simulink subsystem "Day3_Scenario_2"  (R2024a)
settings: Solver=VariableStepAuto  StartTime=0.0  StopTime=10.0  RelTol=1e-3
libraries: CarMaker4SL x8
settings Model: Creator=junhyung.cha  LastModifiedBy=User

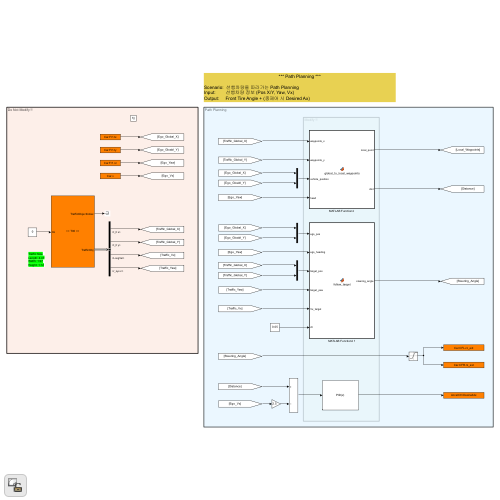
[thumbnail: Simulink's stored preview of the top-level diagram]
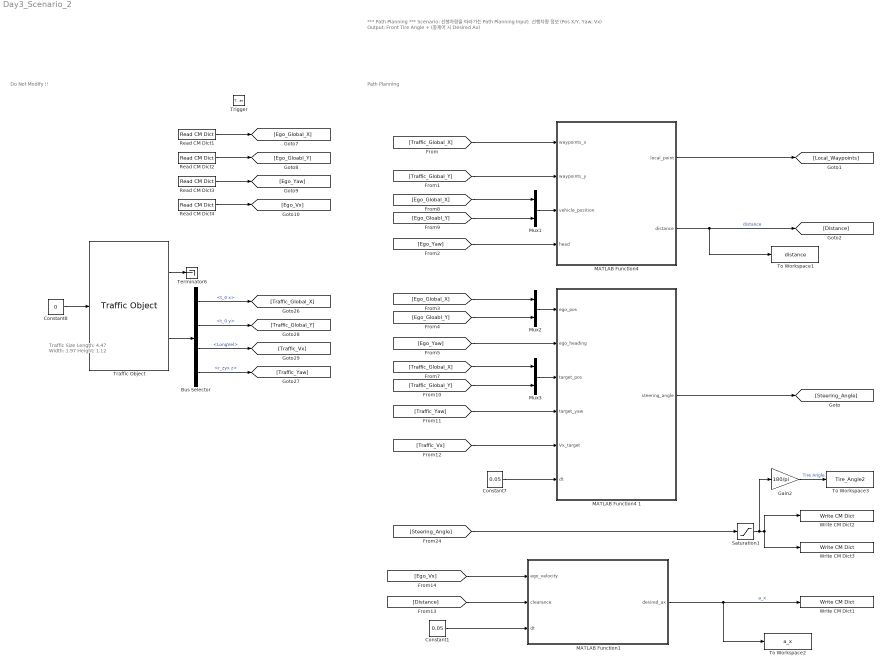
== system Day3_Scenario_2 ==
  note: Path Planning
  note: Do Not Modify !!
  note: *** Path Planning ***
      |
      | Scenario: 선행차량을 따라가는 Path Planning
      | Input: 선행차량 정보 (Pos X/Y, Yaw, Vx)
      | Output: Front Tire Angle + (종제어 시 Desired Ax)
  note: Traffic Size
      | Length: 4.47
      | Width: 1.97
      | Height: 1.12
  Trigger : TriggerPort  TriggerType=function-call  VariantControl=(inherit)
  Bus Selector : BusSelector  OutputSignals=t_0 x,t_0 y,LongVel,r_zyx z
  Constant1 : Constant  Value=0.05
  Constant7 : Constant  Value=0.05
  Constant8 : Constant  Value=0
  Gain2 : Gain  Gain=180/pi
  MATLAB Function1 : MATLAB Function  TreatAsAtomicUnit=on
  "MATLAB Function4 " : MATLAB Function  TreatAsAtomicUnit=on
  MATLAB Function4 1 : MATLAB Function  TreatAsAtomicUnit=on
  Mux1 : Mux  Inputs=2
  Mux2 : Mux  Inputs=2
  Mux3 : Mux  Inputs=2
  Read CM Dict1 : CarMaker4SL/Read CM Dict  xname=Car.Fr1.tx  xsync=off  xstime=Inherited
  Read CM Dict2 : CarMaker4SL/Read CM Dict  xname=Car.Fr1.ty  xsync=off  xstime=Inherited
  Read CM Dict3 : CarMaker4SL/Read CM Dict  xname=Car.Fr1.rz  xsync=off  xstime=Inherited
  Read CM Dict4 : CarMaker4SL/Read CM Dict  xname=Car.v  xsync=off  xstime=Inherited
  Saturation1 : Saturate  UpperLimit=pi/6  LowerLimit=-pi/6
  Terminator6 : Terminator
  To Workspace1 : ToWorkspace  VariableName=distance  SaveFormat=Timeseries  SampleTime=-1
  To Workspace2 : ToWorkspace  VariableName=a_x  SaveFormat=Timeseries  SampleTime=-1
  To Workspace3 : ToWorkspace  VariableName=Tire_Angle2  SaveFormat=Timeseries  SampleTime=-1
  Traffic Object : CarMaker4SL/Traffic Object  xname=T00  ximode=Traffic Id  xstime=Inherited
      settings: SourceProductName=CarMaker4SL
  Write CM Dict1 : CarMaker4SL/Write CM Dict  xname=AccelCtrl.DesiredAx  xsync=off
  Write CM Dict2 : CarMaker4SL/Write CM Dict  xname=Car.CFL.rz_ext  xsync=off
  Write CM Dict3 : CarMaker4SL/Write CM Dict  xname=Car.CFR.rz_ext  xsync=off
  wires:
  Read CM Dict4/1 -> [Ego_Vx]
  Read CM Dict3/1 -> [Ego_Yaw]
  Read CM Dict1/1 -> [Ego_Global_X]
  Read CM Dict2/1 -> [Ego_Gloabl_Y]
  [Steering_Angle] -> Saturation1/1
  Traffic Object/2 -> Bus Selector/1
  Constant8/1 -> Traffic Object/1
  Bus Selector/4 -> [Traffic_Yaw]  "<r_zyx z>"
  Bus Selector/3 -> [Traffic_Vx]  "<LongVel>"
  Traffic Object/1 -> Terminator6/1
  Bus Selector/2 -> [Traffic_Global_Y]  "<t_0 y>"
  Bus Selector/1 -> [Traffic_Global_X]  "<t_0 x>"
  [Traffic_Global_X] -> "MATLAB Function4 "/1(waypoints_x)
  [Traffic_Global_Y] -> "MATLAB Function4 "/2(waypoints_y)
  [Ego_Gloabl_Y] -> Mux1/2
  Mux1/1 -> "MATLAB Function4 "/3(vehicle_position)
  [Ego_Global_X] -> Mux1/1
  [Ego_Yaw] -> "MATLAB Function4 "/4(head)
  "MATLAB Function4 "/1(local_point) -> [Local_Waypoints]
  "MATLAB Function4 "/2(distance) -> [Distance], To Workspace1/1  "distance"
  [Ego_Global_X] -> Mux2/1
  [Ego_Gloabl_Y] -> Mux2/2
  Mux2/1 -> MATLAB Function4 1/1(ego_pos)
  [Ego_Yaw] -> MATLAB Function4 1/2(ego_heading)
  [Traffic_Global_X] -> Mux3/1
  [Traffic_Global_Y] -> Mux3/2
  [Traffic_Yaw] -> MATLAB Function4 1/4(target_yaw)
  Mux3/1 -> MATLAB Function4 1/3(target_pos)
  [Traffic_Vx] -> MATLAB Function4 1/5(Vx_target)
  Constant7/1 -> MATLAB Function4 1/6(dt)
  MATLAB Function4 1/1(steering_angle) -> [Steering_Angle]
  [Ego_Vx] -> MATLAB Function1/1(ego_velocity)
  MATLAB Function1/1(desired_ax) -> Write CM Dict1/1, To Workspace2/1  "a_x"
  Saturation1/1 -> Write CM Dict3/1, Write CM Dict2/1, Gain2/1
  Gain2/1 -> To Workspace3/1  "Tire Angle"
  [Distance] -> MATLAB Function1/2(clearance)
  Constant1/1 -> MATLAB Function1/3(dt)

== matlab function Day3_Scenario_2/MATLAB Function1 ==
  settings: sampleTime=0.05
  data: ego_velocity input; desired_ax output; clearance input; dt input
function desired_ax = longitudinal_variant_space_pd_controller_(ego_velocity, clearance, dt)
    desired_ax = longitudinal_variant_space_pd_controller_mfile(ego_velocity, clearance, dt);
end


function desired_ax = longitudinal_variant_space_pd_controller_mfile(ego_velocity, clearance, dt)
    
    persistent error_prev
    time_gap = 5.0;
    target_distance = ego_velocity*time_gap;

    error = clearance - target_distance;
    
    if isempty(error_prev)
        error_prev = error;
    end

    Kp = 3.0;
    Kd = 1.0;

    P_term = Kp*error;
    D_term = Kd*(error - error_prev) / dt;
    
    desired_ax = (P_term + D_term);
    error_prev = error;
end

== matlab function Day3_Scenario_2/MATLAB Function4  ==
  settings: sampleTime=0.1
  data: waypoints_x input; waypoints_y input; local_point output; vehicle_position input; head input; distance output
function [local_point,distance]  = global_to_local_waypoints_Day3_Scenario_2(waypoints_x,waypoints_y, vehicle_position, head)
    [local_point,distance] = global_to_local_waypoints_Day3_Scenario_2_mfile(waypoints_x,waypoints_y, vehicle_position, head);
end

function [local_point,distance] = global_to_local_waypoints_Day3_Scenario_2_mfile(waypoints_x,waypoints_y, vehicle_position, head)

    vehicle_position = vehicle_position(:)';

    dx = waypoints_x - vehicle_position(1);
    dy = waypoints_y - vehicle_position(2);

    R_inv = [ cos(head),  sin(head);
             -sin(head),  cos(head) ];

    local_point = (R_inv * [dx; dy])';

    distance = sqrt(dx^2 + dy^2);

end

== matlab function Day3_Scenario_2/MATLAB Function4 1 ==
  settings: sampleTime=0.1
  data: ego_pos input; ego_heading input; steering_angle output; target_pos input; target_yaw input; Vx_target input; dt input
function steering_angle = follow_target(ego_pos, ego_heading, target_pos, target_yaw, Vx_target, dt)
    steering_angle = follow_target_mfile(ego_pos, ego_heading, target_pos, target_yaw, Vx_target, dt);
end


function steering_angle = follow_target_mfile(ego_pos, ego_heading, target_pos, target_yaw, Vx_target, dt)

    max_history = 20;
    ego_pos     = ego_pos(:)';
    wheelBase   = 3.85 - 0.95;      
    Ld_gain     = 0.2;       
    Ld_min      = 2.0;       
    Ld_max      = 8.0;       

    persistent localPosArray idx
    
    if isempty(localPosArray)
        localPosArray = zeros(max_history, 2);
        idx = 1;
    end

    R_inv = [cos(ego_heading) sin(ego_heading);
            -sin(ego_heading) cos(ego_heading)];

    dx0 = target_pos(1) - ego_pos(1);
    dy0 = target_pos(2) - ego_pos(2);

    local0 = R_inv * [dx0; dy0];
    x0 = local0(1);
    y0 = local0(2);

    localPosArray(idx, :) = [x0, y0];

    idx = idx + 1;
    if idx > max_history
        idx = 1;
    end

    if nnz(localPosArray(:,1)) < 3
        steering_angle = 0;
        return;
    end

    i2 = idx - 1; if i2 < 1, i2 = max_history; end
    i1 = i2 - 1;  if i1 < 1, i1 = max_history; end

    p1 = localPosArray(i1, :);
    p2 = localPosArray(i2, :);

    dx_h = p2(1) - p1(1);
    dy_h = p2(2) - p1(2);

    heading_local = atan2(dy_h, dx_h);

    x_forward = 0 : 0.1 : 15;
    N = length(x_forward);

    future_points = zeros(N, 2);
    last_pos = p2;

    for k = 1:N
        dx_f = x_forward(k);
        future_points(k,1) = last_pos(1) + dx_f * cos(heading_local);
        future_points(k,2) = last_pos(2) + dx_f * sin(heading_local);
    end

    Ld = max(Ld_min, min(Ld_max, Ld_gain * Vx_target));


    dist_list = sqrt(future_points(:,1).^2 + future_points(:,2).^2);
    [~, idx_Ld] = min(abs(dist_list - Ld));

    yL = future_points(idx_Ld, 2);

    steering_angle = atan2(2 * wheelBase * yL, Ld^2);

end
